simulink library "passthrough"  (Simulink 7.6)
settings: Solver=ode45  SolverMode=SingleTasking  StartTime=0.0  StopTime=10.0  RelTol=1e-3
undefined symbols (not defined in the file or in its folder): passThroughSelector
libraries: passthrough x1
settings Model: Creator=The MathWorks Inc.

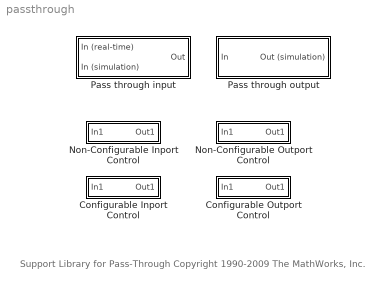
== system passthrough ==
  note: Support Library for Pass-Through
      | Copyright 1990-2009 The MathWorks, Inc.
  Configurable Inport Control : Subsystem  mask(Configurable Inport Control){portNum=1, portName=MyConfigurableInport, isEnabled=1, isConfigurable=1, isInport=1}
      mask prompts: portNum "Port number (when ALL ports are enabled):"; portName "Port name:"; isEnabled "Enabled?:"; isConfigurable "Configurable?:"; isInport "Inport?:"
      mask help: Add this block to a signal immediately after an Inport to specify that this is a configurable Inport. The associated Inport can be selectively controlled by providing the Port Name parameter to the Simulink port control utility. The Port Number parameter will provide the desired Port Number of the Inport when all Inports are enabled.
      mask init:
      | switch (isEnabled)
      | 	case 0 % disabled
      | 		state = 'Disabled';
      | 	case 1 % enabled
      | 		state = 'Enabled';
      | end;
      | dispstr = [num2str(portNum) ' : ' state];
      mask Display: disp(dispstr);
  Configurable Outport Control : Subsystem  mask(Configurable Outport Control){portNum=1, portName=MyConfigurableOutport, isEnabled=1, isConfigurable=1, isInport=0}
      mask prompts: portNum "Port number (when ALL ports are enabled):"; portName "Port name:"; isEnabled "Enabled?:"; isConfigurable "Configurable?:"; isInport "Inport?:"
      mask help: Add this block to a signal immediately before an Outport to specify that this is a configurable Outport. The associated Outport can be selectively controlled by providing the Port Name parameter to the Simulink port control utility. The Port Number parameter will provide the desired Port Number of the Outport when all Outports are enabled.
      mask init:
      | switch (isEnabled)
      | 	case 0 % disabled
      | 		state = 'Disabled';
      | 	case 1 % enabled
      | 		state = 'Enabled';
      | end;
      | dispstr = [state ' : ' num2str(portNum)];
      mask Display: disp(dispstr);
  Non-Configurable Inport Control : Subsystem  mask(Non-Configurable Inport Control){portNum=1, isEnabled=1, isConfigurable=0, isInport=1}
      mask prompts: portNum "Port number (when ALL ports are enabled):"; isEnabled "Enabled?:"; isConfigurable "Configurable?:"; isInport "Inport?:"
      mask help: Add this block to a signal immediately after an Inport to specify that this is a non-configurable Inport. The associated Inport will always be enabled. The Port Number parameter will provide the desired Port Number of the Inport when all Inports are enabled.
      mask Display: disp(['Inport ' num2str(portNum)]);
  Non-Configurable Outport Control : Subsystem  mask(Non-Configurable Outport Control){portNum=1, isEnabled=1, isConfigurable=0, isInport=0}
      mask prompts: portNum "Port number (when ALL ports are enabled):"; isEnabled "Enabled:"; isConfigurable "Configurable?:"; isInport "Inport?:"
      mask help: Add this block to a signal immediately before an Outport to specify that this is a non-configurable Outport. The associated Outport will always be enabled. The Port Number parameter will provide the desired Port Number of the Outport when all Outports are enabled.
      mask Display: disp(['Outport ' num2str(portNum)]);
  Pass through input : Subsystem
      mask Type: Simulation pass through (input)
      mask Description:
      | Pass through input 1 during real-time code generation.
      | Pass through input 2 during simulation and when generating code for simulation (e.g., Accelerator, S-Function target, Processor-in-the-loop).
  Pass through output : Subsystem  mask(Simulation pass through (output)){driverBlock=gcs}
      mask prompts: driverBlock "Driver block reference:"
      mask help:
      | Pass through input during simulation and when generating code for simulation (e.g., Accelerator, S-Function target, Processor-in-the-loop). When generating real-time code the output of this block is not generated.
      |
      | The port width must not be -1
      mask init:
      | % remove \n's from driver block
      | driverBlock = regexprep(driverBlock, sprintf('\n'), ' ');
      | % get the closest target subsystem to the driver block
      | targetSubsystem = RTWConfigurationCB('get_target_subsystem', driverBlock);
      | % check the pass through output
      | passThroughOutputChecker(gcb, driverBlock, targetSubsystem, 0);

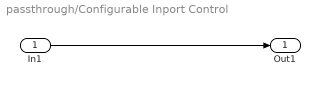
== system passthrough/Configurable Inport Control ==
  In1 : Inport
  Out1 : Outport
  wires:
  In1/1 -> Out1/1

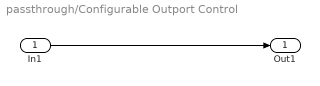
== system passthrough/Configurable Outport Control ==
  In1 : Inport
  Out1 : Outport
  wires:
  In1/1 -> Out1/1

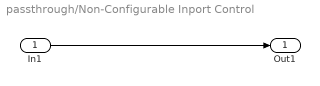
== system passthrough/Non-Configurable Inport Control ==
  In1 : Inport
  Out1 : Outport
  wires:
  In1/1 -> Out1/1

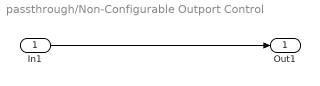
== system passthrough/Non-Configurable Outport Control ==
  In1 : Inport
  Out1 : Outport
  wires:
  In1/1 -> Out1/1

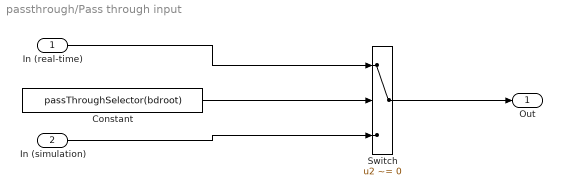
== system passthrough/Pass through input ==
  In (real-time) : Inport
  In (simulation) : Inport  Port=2
  Constant : Constant  Value=passThroughSelector(bdroot)  OutDataTypeStr=boolean
  Switch : Switch  Criteria=u2 ~= 0  SaturateOnIntegerOverflow=on  InputSameDT=on
  Out : Outport
  wires:
  In (real-time)/1 -> Switch/1
  Constant/1 -> Switch/2
  In (simulation)/1 -> Switch/3
  Switch/1 -> Out/1

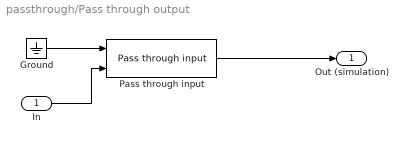
== system passthrough/Pass through output ==
  In : Inport
  Ground : Ground
  Pass through input : passthrough/Pass through input
  Out (simulation) : Outport
  wires:
  Ground/1 -> Pass through input/1
  In/1 -> Pass through input/2
  Pass through input/1 -> Out (simulation)/1
